simulink model "gamingJoystick"  (Simulink 10.0)
settings: Solver=ode23tb  StartTime=0.0  StopTime=1000.0  MaxStep=1  RelTol=1e-3  EnableMultiTasking=on
libraries: LemmingToolbox x11
settings Model: Creator=langmo  LastModifiedBy=unknown
settings DataIOCC: LimitDataPoints=on  SignalLoggingSaveFormat=ModelDataLogs
settings OptimizationCC: ExpressionDepthLimit=2147483647  InitFltsAndDblsToZero=on
settings DebuggingCC: SolverPrmCheckMsg=warning  FcnCallInpInsideContextMsg=warning  StateNameClashWarn=warning
settings SFSimCC: SimUseLocalCustomCode=on  CustomCodeUndefinedFunction=FilterOut
settings RTWCC: RTWUseLocalCustomCode=on

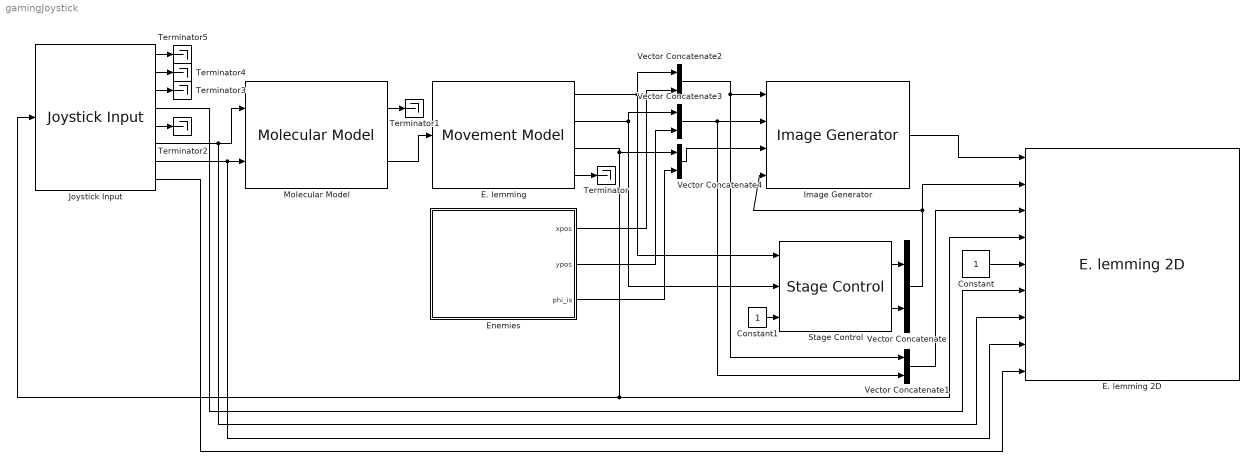
== system gamingJoystick ==
  Constant : Constant  OutDataTypeStr=uint32
  Constant1 : Constant
  E. lemming : LemmingToolbox/Movement Model  imageDim=[1344,1024]  binning=2  pixelSize=6.45 / 40  initialCondition=[0.5, 0.5, 0]  sampleTimes=[0.03, 0]
  E. lemming 2D : LemmingToolbox/E. lemming 2D  SystemSampleTime=-1  outputFilename=game.avi  imageDim=[1344,1024]  binning=2  maxNumCells=6  coneWidth=150  coneAngle=pi/4  pathLength=30  sampleTimes=[0.3, 0.1]
  Enemies : Subsystem
  Image Generator : LemmingToolbox/Image Generator  binning=2  numCells=6  sampleTime=[0.3, 0.1]
  Joystick Input : LemmingToolbox/Joystick Input  SystemSampleTime=1  minMaxThresh=[0.05, 0.2]  sampleTimes=[0.1, 0]
  Molecular Model : LemmingToolbox/Molecular Model  molecModel=Spiro  controlledCheSpecies=CheY  cheSpeciesAttachedTo=CheX-PhyB & PIF3-Anker  asp=1e-3  useOrgParameters=off  CheX=40  AnkerProt=60  Anker=80
  Stage Control : LemmingToolbox/Stage Control  SystemSampleTime=-1  activate=on  controlMicroscope=off  cooldown=0  border=0.25  initialCondition=[0, 0]  sampleTimes=[0.3, 0.1]
  Terminator{,1..5} (6 alike) : Terminator
  Vector Concatenate : Concatenate  ConcatenateDimension=2
  Vector Concatenate1 : Concatenate  Mode=Multidimensional array  ConcatenateDimension=2
  Vector Concatenate2 : Concatenate
  Vector Concatenate3 : Concatenate
  Vector Concatenate4 : Concatenate
  wires:
  Stage Control/2 -> Vector Concatenate/2
  Stage Control/1 -> Vector Concatenate/1
  Joystick Input/6 -> Molecular Model/1, E. lemming 2D/7
  Molecular Model/2 -> E. lemming/1
  E. lemming/1 -> Vector Concatenate2/1, Stage Control/1
  E. lemming/2 -> Vector Concatenate3/1, Stage Control/2
  E. lemming/3 -> E. lemming 2D/4, Joystick Input/1, Vector Concatenate4/1
  Vector Concatenate/1 -> Image Generator/4, E. lemming 2D/2
  Joystick Input/4 -> E. lemming 2D/6
  Image Generator/1 -> E. lemming 2D/1
  Vector Concatenate1/1 -> E. lemming 2D/3
  Constant/1 -> E. lemming 2D/5
  E. lemming/4 -> Terminator/1
  Molecular Model/1 -> Terminator1/1
  Joystick Input/5 -> Terminator2/1
  Joystick Input/3 -> Terminator3/1
  Joystick Input/2 -> Terminator4/1
  Joystick Input/1 -> Terminator5/1
  Joystick Input/7 -> Molecular Model/2, E. lemming 2D/8
  Constant1/1 -> Stage Control/3
  Joystick Input/8 -> E. lemming 2D/9
  Vector Concatenate2/1 -> Image Generator/1, Vector Concatenate1/1
  Vector Concatenate3/1 -> Image Generator/2, Vector Concatenate1/2
  Vector Concatenate4/1 -> Image Generator/3
  Enemies/1(xpos) -> Vector Concatenate2/2
  Enemies/2(ypos) -> Vector Concatenate3/2
  Enemies/3(phi_is) -> Vector Concatenate4/2

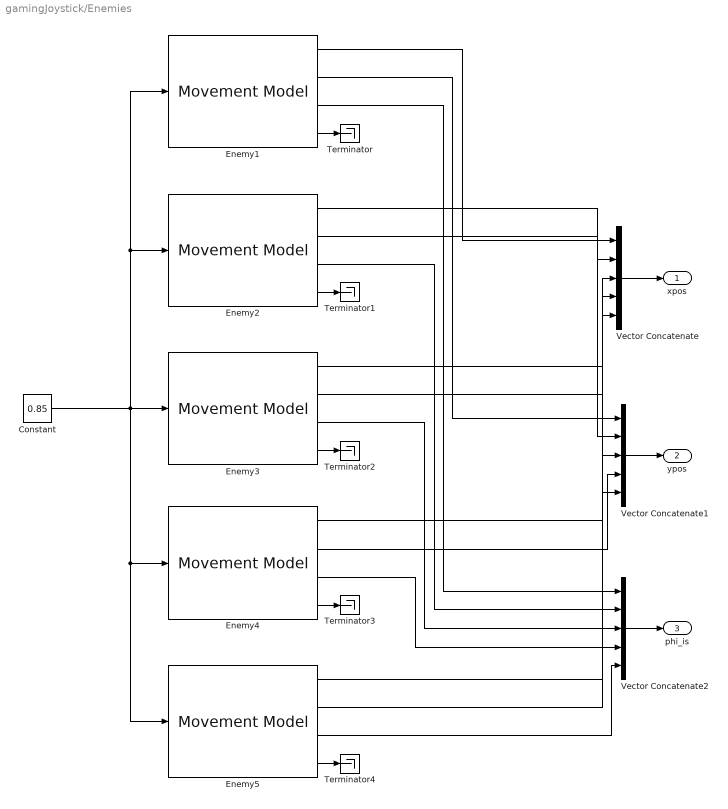
== system gamingJoystick/Enemies ==
  Constant : Constant  Value=0.85
  Enemy1 : LemmingToolbox/Movement Model  imageDim=[1344,1024]  binning=2  pixelSize=6.45 / 40  initialCondition=[0.1, 0.2, 0]  sampleTimes=[0.03, 0]
  Enemy2 : LemmingToolbox/Movement Model  imageDim=[1344,1024]  binning=2  pixelSize=6.45 / 40  initialCondition=[0.8, 0.1, 0]  sampleTimes=[0.03, 0]
  Enemy3 : LemmingToolbox/Movement Model  imageDim=[1344,1024]  binning=2  pixelSize=6.45 / 40  initialCondition=[0.5, 0.9, 0]  sampleTimes=[0.03, 0]
  Enemy4 : LemmingToolbox/Movement Model  imageDim=[1344,1024]  binning=2  pixelSize=6.45 / 40  initialCondition=[0.7, 0.3, 0]  sampleTimes=[0.03, 0]
  Enemy5 : LemmingToolbox/Movement Model  imageDim=[1344,1024]  binning=2  pixelSize=6.45 / 40  initialCondition=[0.3, 0.6, 0]  sampleTimes=[0.03, 0]
  Terminator{,1..4} (5 alike) : Terminator
  Vector Concatenate : Concatenate  NumInputs=5
  Vector Concatenate1 : Concatenate  NumInputs=5
  Vector Concatenate2 : Concatenate  NumInputs=5
  xpos : Outport
  ypos : Outport  Port=2
  phi_is : Outport  Port=3
  wires:
  Vector Concatenate/1 -> xpos/1
  Vector Concatenate1/1 -> ypos/1
  Vector Concatenate2/1 -> phi_is/1
  Enemy1/1 -> Vector Concatenate/1
  Enemy1/2 -> Vector Concatenate1/1
  Enemy1/3 -> Vector Concatenate2/1
  Enemy2/1 -> Vector Concatenate/2
  Enemy2/2 -> Vector Concatenate1/2
  Enemy2/3 -> Vector Concatenate2/2
  Enemy3/1 -> Vector Concatenate/3
  Enemy3/2 -> Vector Concatenate1/3
  Enemy3/3 -> Vector Concatenate2/3
  Enemy4/1 -> Vector Concatenate/4
  Enemy4/2 -> Vector Concatenate1/4
  Enemy4/3 -> Vector Concatenate2/4
  Enemy5/1 -> Vector Concatenate/5
  Enemy5/2 -> Vector Concatenate1/5
  Enemy5/3 -> Vector Concatenate2/5
  Constant/1 -> Enemy3/1, Enemy4/1, Enemy5/1, Enemy2/1, Enemy1/1
  Enemy1/4 -> Terminator/1
  Enemy2/4 -> Terminator1/1
  Enemy3/4 -> Terminator2/1
  Enemy4/4 -> Terminator3/1
  Enemy5/4 -> Terminator4/1
